simulink model "Simulink_VDP_KK"  (R2022a)
settings: Solver=FixedStepAuto  StartTime=0.0  StopTime=Tf  FixedStep=Ts  RelTol=1e-3
values from neighbouring files (symbols this model uses):
  A_kalman = A    [VanDerPol_MPC_Evaluation.m]
  B_kalman = B    [VanDerPol_MPC_Evaluation.m]
  D = zeros(size(Z,1),size(U,1))    [VanDerPol_MPC_Koopman.m]
  eta = 0.001    [VanDerPol_MPC.m]    (also in VanDerPol_MPC_Evaluation.m)
  kalman_0 = Spline_Radial_Obs([0;0],X0_kalman)    [VanDerPol_MPC_Evaluation.m]
  Tf = 2e3    (= 2000)    [VanDerPol_MPC.m]    (also in VanDerPol_MPC_Evaluation.m = 20)
  Ts = 1e-2    (= 0.01)    [VanDerPol_MPC.m]
undefined symbols (not defined in the file or in its folder): A, B
libraries: sharedTrackingLibrary x1, mpclib x1
settings Model: Creator=sergiovaneg  LastModifiedBy=sergiovaneg

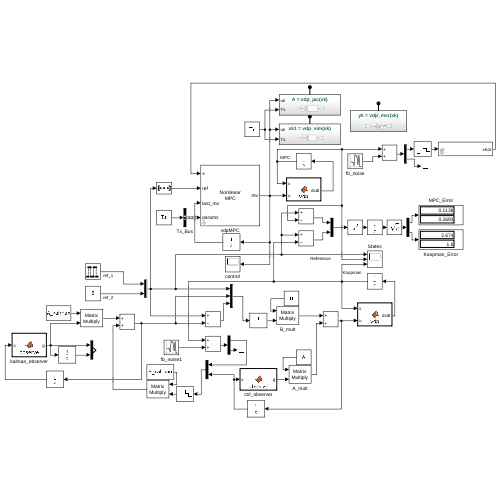
[thumbnail: Simulink's stored preview of the top-level diagram]
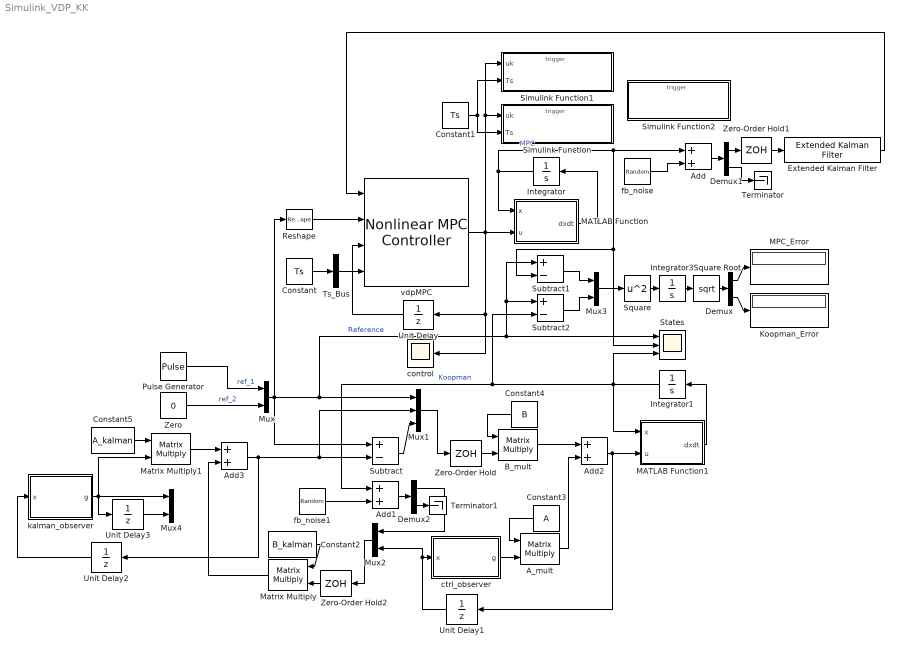
== system Simulink_VDP_KK ==
  A_mult : Product  Multiplication=Matrix(*)
  Add{,1..3} (4 alike) : Sum
  B_mult : Product  Multiplication=Matrix(*)
  Constant : Constant  Value=Ts
  Constant1 : Constant  Value=Ts
  Constant2 : Constant  Value=B_kalman  VectorParams1D=off
  Constant3 : Constant  Value=A  VectorParams1D=off
  Constant4 : Constant  Value=B  VectorParams1D=off
  Constant5 : Constant  Value=A_kalman  VectorParams1D=off
  Demux : Demux  Outputs=2
  Demux1 : Demux  Outputs=2
  Demux2 : Demux  Outputs=2
  Extended Kalman Filter : sharedTrackingLibrary/Extended Kalman Filter  StateTransitionFcn=vdp_sim  HasStateTransitionJacobianFcn=on  StateTransitionJacobianFcn=vdp_jac  HasAdditiveProcessNoise=Additive  ProcessNoise=0  HasTimeVaryingProcessNoise=off  HasStateTransitionFcnExtraArgument=0  InitialState=[0;0]  InitialStateCovariance=eta  MeasurementFcn1=vdp_msr  HasMeasurementJacobianFcn1=off  HasMeasurementEnablePort1=off  HasAdditiveMeasurementNoise1=Additive  MeasurementNoise1=eta  HasTimeVaryingMeasurementNoise1=off  HasMeasurementFcnExtraArgument1=0  HasMeasurementWrapping1=off  MeasurementFcn2=myMeasurementFcn  HasMeasurementJacobianFcn2=off  HasMeasurementEnablePort2=off  HasAdditiveMeasurementNoise2=Additive  MeasurementNoise2=1  HasTimeVaryingMeasurementNoise2=off  HasMeasurementFcnExtraArgument2=0  HasMeasurementWrapping2=off  MeasurementFcn3=myMeasurementFcn  HasMeasurementJacobianFcn3=off  HasMeasurementEnablePort3=off  HasAdditiveMeasurementNoise3=Additive  MeasurementNoise3=1  HasTimeVaryingMeasurementNoise3=off  HasMeasurementFcnExtraArgument3=0  HasMeasurementWrapping3=off  MeasurementFcn4=myMeasurementFcn  HasMeasurementJacobianFcn4=off  HasMeasurementEnablePort4=off  HasAdditiveMeasurementNoise4=Additive  MeasurementNoise4=1  HasTimeVaryingMeasurementNoise4=off  HasMeasurementFcnExtraArgument4=0  HasMeasurementWrapping4=off  MeasurementFcn5=myMeasurementFcn  HasMeasurementJacobianFcn5=off  HasMeasurementEnablePort5=off  HasAdditiveMeasurementNoise5=Additive  MeasurementNoise5=1  HasTimeVaryingMeasurementNoise5=off  HasMeasurementFcnExtraArgument5=0  HasMeasurementWrapping5=off  EnableMultirate=off  StateTransitionFcnSampleTime=1  MeasurementFcn1SampleTime=1  MeasurementFcn2SampleTime=1  MeasurementFcn3SampleTime=1  MeasurementFcn4SampleTime=1  MeasurementFcn5SampleTime=1  UseCurrentEstimator=on  OutputStateCovariance=off  DataType=double  SampleTime=Ts  NumberOfMeasurements=1
      settings: SourceProductBaseCode=TF,AE,PW,CT,DR,ID,LP,NV,AR,RO,RR,UV,VE
  Integrator : Integrator  InitialCondition=[0;0]
  Integrator1 : Integrator  InitialCondition=[0;0]
  Integrator3 : Integrator
  Koopman_Error : Display
  MATLAB Function : MATLAB Function  TreatAsAtomicUnit=on
  MATLAB Function1 : MATLAB Function  TreatAsAtomicUnit=on
  MPC_Error : Display
      settings: Decimation=3
  Matrix Multiply : Product  Multiplication=Matrix(*)
  Matrix Multiply1 : Product  Multiplication=Matrix(*)
  Mux{,2..4} (4 alike) : Mux  Inputs=2
  Mux1 : Mux  Inputs=3
  Pulse Generator : DiscretePulseGenerator  Period=Tf/Ts+1  SampleTime=Ts
  Reshape : Reshape  OutputDimensionality=Row vector (2-D)
  Simulink Function : Subsystem  TreatAsAtomicUnit=on
  Simulink Function1 : Subsystem  TreatAsAtomicUnit=on
  Simulink Function2 : Subsystem  TreatAsAtomicUnit=on
  Square : Math  Operator=square
  Square Root : Sqrt
  States : Scope  NumInputPorts=3
  Subtract : Sum  Inputs=+-
  Subtract1 : Sum  Inputs=+-
  Subtract2 : Sum  Inputs=+-
  Terminator : Terminator
  Terminator1 : Terminator
  Ts_Bus : BusCreator  Inputs=1  OutDataTypeStr=Bus: Ts_Bus  NonVirtualBus=on
      settings: InheritFromInputs=off
  Unit Delay : UnitDelay  SampleTime=-1  HasFrameUpgradeWarning=on
  Unit Delay1 : UnitDelay  SampleTime=Ts  HasFrameUpgradeWarning=on
  Unit Delay2 : UnitDelay  InitialCondition=[0;0]  SampleTime=Ts  HasFrameUpgradeWarning=on
  Unit Delay3 : UnitDelay  InitialCondition=kalman_0  SampleTime=Ts  HasFrameUpgradeWarning=on
  Zero : Constant  Value=0  OutDataTypeStr=Inherit: Inherit via back propagation
  Zero-Order Hold : ZeroOrderHold  SampleTime=Ts
  Zero-Order Hold1 : ZeroOrderHold  SampleTime=Ts
  Zero-Order Hold2 : ZeroOrderHold  SampleTime=Ts
  control : Scope
  ctrl_observer : MATLAB Function  TreatAsAtomicUnit=on
  fb_noise : RandomNumber  Variance=eta  Seed=[2;3]  SampleTime=Ts
  fb_noise1 : RandomNumber  Variance=eta  Seed=[2;3]  SampleTime=Ts
  kalman_observer : MATLAB Function  TreatAsAtomicUnit=on
  vdpMPC : mpclib/Nonlinear MPC Controller  nlmpcobj=nlobj  UseObjectTs=on  UseMEX=off  md_enabled=off  mvtarget_enabled=off  param_enabled=on  cost_enabled=off  mvseq_enabled=off  stateseq_enabled=off  ovseq_enabled=off  slack_enabled=off  status_enabled=off  ov_min=off  ov_max=off  mv_min=off  mv_max=off  mvrate_min=off  mvrate_max=off  state_min=off  state_max=off  ov_weight=off  mv_weight=off  mvrate_weight=off  ecr_weight=off  nlp_initialize=off
  wires:
  Pulse Generator/1 -> Mux/1  "ref_1"
  Integrator/1 -> Add/1, Subtract1/2, States/2, MATLAB Function/1(x)  "MPC"
  Zero/1 -> Mux/2  "ref_2"
  Mux/1 -> Subtract/1, Subtract1/1, Subtract2/1, States/1, Mux1/1, Reshape/1  "Reference"
  Integrator1/1 -> States/3, Add1/1, Subtract2/2, MATLAB Function1/1(x)  "Koopman"
  Add2/1 -> Unit Delay1/1, MATLAB Function1/2(u)
  MATLAB Function/1(dxdt) -> Integrator/1
  vdpMPC/1 -> Simulink Function1/1(uk), Simulink Function/1(uk), Unit Delay/1, control/1, MATLAB Function/2(u)
  MATLAB Function1/1(dxdt) -> Integrator1/1
  Constant/1 -> Ts_Bus/1
  A_mult/1 -> Add2/2
  Constant4/1 -> B_mult/1
  Constant3/1 -> A_mult/1
  Unit Delay/1 -> vdpMPC/3
  B_mult/1 -> Add2/1
  Reshape/1 -> vdpMPC/2
  Unit Delay1/1 -> Mux2/2, ctrl_observer/1(x)
  Ts_Bus/1 -> vdpMPC/4
  fb_noise1/1 -> Add1/2
  Mux1/1 -> Zero-Order Hold/1
  Subtract/1 -> Mux1/3
  Subtract1/1 -> Mux3/1
  Subtract2/1 -> Mux3/2
  Mux3/1 -> Square/1
  Square/1 -> Integrator3/1
  Integrator3/1 -> Square Root/1
  Square Root/1 -> Demux/1
  Demux/1 -> MPC_Error/1
  Demux/2 -> Koopman_Error/1
  fb_noise/1 -> Add/2
  Constant1/1 -> Simulink Function1/2(Ts), Simulink Function/2(Ts)
  Extended Kalman Filter/1 -> vdpMPC/1
  Add/1 -> Demux1/1
  Demux1/2 -> Terminator/1
  Demux1/1 -> Zero-Order Hold1/1
  Zero-Order Hold1/1 -> Extended Kalman Filter/1
  Add1/1 -> Demux2/1
  Demux2/2 -> Terminator1/1
  Zero-Order Hold/1 -> B_mult/2
  ctrl_observer/1(g) -> A_mult/2
  Zero-Order Hold2/1 -> Matrix Multiply/2
  Constant2/1 -> Matrix Multiply/1
  Demux2/1 -> Mux2/1
  Mux2/1 -> Zero-Order Hold2/1
  Constant5/1 -> Matrix Multiply1/1
  Add3/1 -> Unit Delay2/1, Mux1/2, Subtract/2
  Matrix Multiply1/1 -> Add3/1
  Matrix Multiply/1 -> Add3/2
  Unit Delay2/1 -> kalman_observer/1(x)
  Unit Delay3/1 -> Mux4/2
  kalman_observer/1(g) -> Matrix Multiply1/2, Mux4/1, Unit Delay3/1

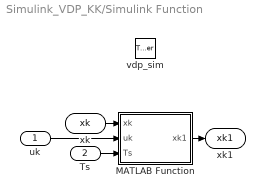
== system Simulink_VDP_KK/Simulink Function ==
  uk : Inport
  Ts : Inport  Port=2
  vdp_sim : TriggerPort  TriggerType=function-call  IsSimulinkFunction=on  FunctionName=vdp_sim  FunctionVisibility=scoped  VariantControl=(inherit)
  MATLAB Function : MATLAB Function  TreatAsAtomicUnit=on
  xk : ArgIn  DisableCoverage=on  PortDimensions=2  ArgumentName=xk
  xk1 : ArgOut  DisableCoverage=on  PortDimensions=2  ArgumentName=xk1
  wires:
  xk/1 -> MATLAB Function/1(xk)
  MATLAB Function/1(xk1) -> xk1/1
  uk/1 -> MATLAB Function/2(uk)
  Ts/1 -> MATLAB Function/3(Ts)

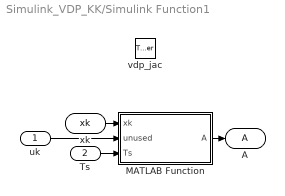
== system Simulink_VDP_KK/Simulink Function1 ==
  uk : Inport
  Ts : Inport  Port=2
  vdp_jac : TriggerPort  TriggerType=function-call  IsSimulinkFunction=on  FunctionName=vdp_jac  FunctionVisibility=scoped  VariantControl=(inherit)
  MATLAB Function : MATLAB Function  TreatAsAtomicUnit=on
  xk : ArgIn  DisableCoverage=on  PortDimensions=2  ArgumentName=xk
  A : ArgOut  DisableCoverage=on  PortDimensions=[2 2]  ArgumentName=A
  wires:
  xk/1 -> MATLAB Function/1(xk)
  MATLAB Function/1(A) -> A/1
  uk/1 -> MATLAB Function/2(unused)
  Ts/1 -> MATLAB Function/3(Ts)

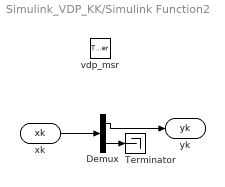
== system Simulink_VDP_KK/Simulink Function2 ==
  vdp_msr : TriggerPort  TriggerType=function-call  IsSimulinkFunction=on  FunctionName=vdp_msr  FunctionVisibility=scoped  VariantControl=(inherit)
  Demux : Demux  Outputs=2
  Terminator : Terminator
  xk : ArgIn  DisableCoverage=on  PortDimensions=2  ArgumentName=xk
  yk : ArgOut  DisableCoverage=on  ArgumentName=yk
  wires:
  xk/1 -> Demux/1
  Demux/1 -> yk/1
  Demux/2 -> Terminator/1

== matlab function Simulink_VDP_KK/MATLAB Function ==
  data: x input; u input; dxdt output
function dxdt = vdp(x,u)
    dxdt = zeros(2,1);
    dxdt(1) = 2*x(2);
    dxdt(2) = -0.8*x(1)+2*x(2)-10*(x(1)^2)*x(2)+u;

== matlab function Simulink_VDP_KK/ctrl_observer ==
  data: x input; g output; X0 parameter
function g = observe(x,X0)
    g=zeros(size(x,1)+size(X0,2),1);
    aux = vecnorm(X0-x)';
    g(1:size(x,1))=x;
    g(size(x,1)+1:end)=aux.*log(aux.^aux);
end

== matlab function Simulink_VDP_KK/Simulink Function/MATLAB Function ==
  data: xk input; xk1 output; uk input; Ts input
function xk1 = vdp(xk,uk,Ts)
    M = 10;

    delta = Ts/M;
    xk1 = xk;
    for ct=1:M
        xk1 = xk1+delta*vdp_CT0(xk,uk);
    end
end

== matlab function Simulink_VDP_KK/Simulink Function1/MATLAB Function ==
  data: xk input; A output; unused input; Ts input
function A = fcn(xk,~,Ts)
    A=[1,2*Ts;
        Ts*(-0.8-20*xk(1)*xk(2)),1+Ts*(2-xk(1)^2)];
end

== matlab function Simulink_VDP_KK/kalman_observer ==
  data: x input; g output; X0_kalman parameter
function g = observe(x,X0_kalman)
    g=zeros(size(x,1)+size(X0_kalman,2),1);
    aux = vecnorm(X0_kalman-x)';
    g(1:size(x,1))=x;
    g(size(x,1)+1:end)=aux.*log(aux.^aux);
end

== matlab function Simulink_VDP_KK/MATLAB Function1 ==
  data: x input; u input; dxdt output
function dxdt = vdp(x,u)
    dxdt = zeros(2,1);
    dxdt(1) = 2*x(2);
    dxdt(2) = -0.8*x(1)+2*x(2)-10*(x(1)^2)*x(2)+u;
